simulink model "MotorXploer"  (R2024b)
settings: Solver=FixedStepAuto  StartTime=0.0  StopTime=inf  FixedStep=0.001  RelTol=1e-3
undefined symbols (not defined in the file): Blocking, LF, Non
libraries: hdlsllib x5, amg_usbconverter_n_connect_lib x3
settings Model: Creator=beamk  LastModifiedBy=pongn

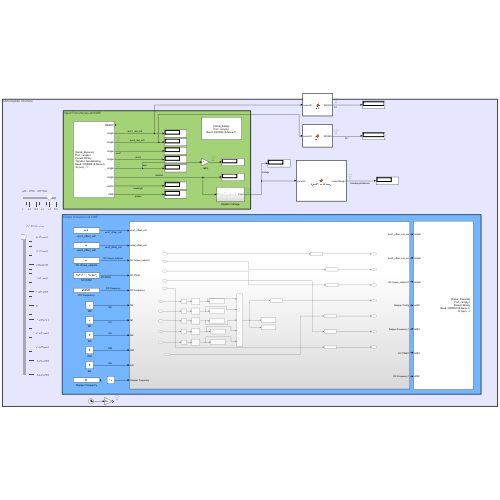
[thumbnail: Simulink's stored preview of the top-level diagram]
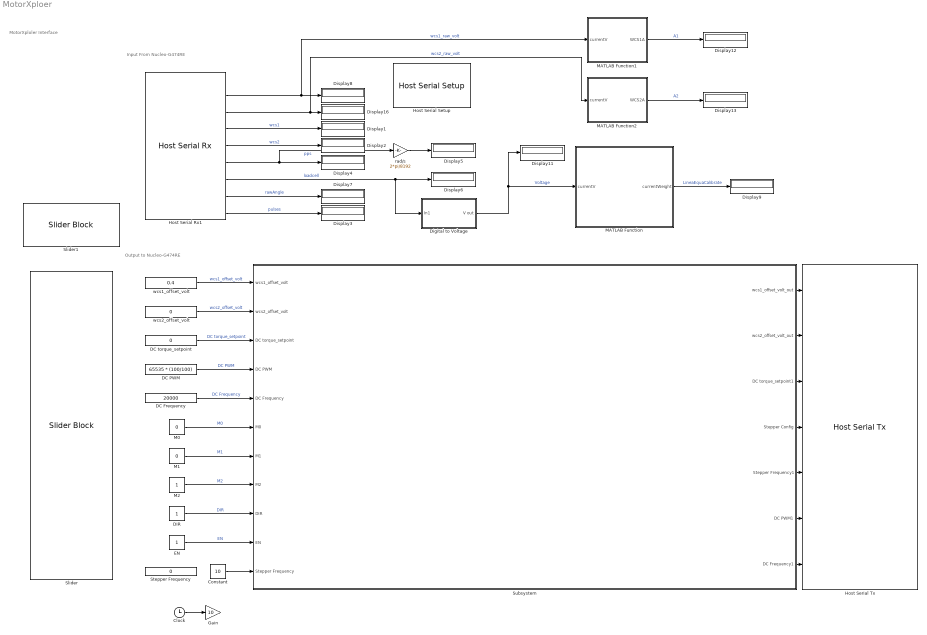
== system MotorXploer ==
  note: Output to Nucleo-G474RE
  note: Input From Nucleo-G474RE
  note: MotorXploler Interface
  Clock : Clock
  Constant : Constant  Value=10
  DC Frequency : Constant  Value=20000
  DC PWM : Constant  Value=65535 * (100/100)
  DC torque_setpoint : Constant  Value=0
  DIR : Constant  OutDataTypeStr=uint8
  Digital to Voltage : Subsystem
  Display{1..9,11..13,16} (13 alike) : Display
  EN : Constant  OutDataTypeStr=uint8
  Gain : Gain  Gain=10
  Host Serial Rx1 : amg_usbconverter_n_connect_lib/Host Serial Rx  conf=rx  port=<auto>  baudrate=2000000  databits=8  parity=None  stopbit=1  flowcontrol=None  transfer=Non-Blocking  timeout=5  packetmode=Binary  enableinitialvalues=off  initialvalues=[]  binheader='45'  binterminator='A'  porttype_double=0  porttype_single=6  porttype_int8=0  porttype_uint8=0  porttype_int16=0  porttype_uint16=1  porttype_int32=1  porttype_uint32=0  asciiformat='%f,%f,%d,%d'  rx_asciiterminator="LF (0x0A - \"\\n\")"  tx_asciiterminator="CRLF (0x0D 0x0A - \"\\r\\n\")"  sampletime=-1  enablecustomportlabel=off  cinputportlabel=0  coutputportlabel=A  portpinstr=0  blockid=HostSerialRx1  inputporttype=[]  inputportwidth=[]  inputportlabel={}  outputporttype=[3 1 1 1 1 1 1 5 6]  outputportwidth=[1 1 1 1 1 1 1 1 1]  outputportlabel={'READY','single','single','single','single','single','single','uint16','int32'}  compat=0  optionstring=[]  autoport='<empty>'
  Host Serial Setup : amg_usbconverter_n_connect_lib/Host Serial Setup  conf=setup  port=<auto>  baudrate=2000000  databits=8  parity=None  stopbit=1  flowcontrol=None  transfer=Blocking  timeout=2  packetmode=Binary  initialvalues=[]  binheader='7E 7E'  binterminator='03 03'  porttype_double=0  porttype_single=1  porttype_int8=0  porttype_uint8=0  porttype_int16=0  porttype_uint16=0  porttype_int32=0  porttype_uint32=2  asciiformat='%d %u %x'  rx_asciiterminator="CRLF (0x0D 0x0A - \"\\r\\n\")"  tx_asciiterminator="CRLF (0x0D 0x0A - \"\\r\\n\")"  sampletime=-1  enablecustomportlabel=off  cinputportlabel=0  coutputportlabel=A  portpinstr=0  blockid=HostSerialSetup  inputporttype=[]  inputportwidth=[]  inputportlabel={}  outputporttype=[]  outputportwidth=[]  outputportlabel={}  compat=0  optionstring=[]  autoport='<empty>'
  Host Serial Tx : amg_usbconverter_n_connect_lib/Host Serial Tx  conf=tx  port=<auto>  baudrate=2000000  databits=8  parity=None  stopbit=1  flowcontrol=None  transfer=Blocking  timeout=2  packetmode=Binary  initialvalues=[]  binheader='45'  binterminator='A'  porttype_double=0  porttype_single=3  porttype_int8=0  porttype_uint8=1  porttype_int16=0  porttype_uint16=0  porttype_int32=3  porttype_uint32=0  asciiformat='%d,%f'  rx_asciiterminator="CRLF (0x0D 0x0A - \"\\r\\n\")"  tx_asciiterminator="CRLF (0x0D 0x0A - \"\\r\\n\")"  sampletime=-1  enablecustomportlabel=off  cinputportlabel=0  coutputportlabel=A  portpinstr=0  blockid=HostSerialTx  inputporttype=[1 1 1 3 6 6 6]  inputportwidth=[1 1 1 1 1 1 1]  inputportlabel={'single','single','single','uint8','int32','int32','int32'}  outputporttype=[]  outputportwidth=[]  outputportlabel={}  compat=0  optionstring=[]  autoport='<empty>'
      settings: SourceProductName=aMG USB Converter N
  M0 : Constant  Value=0  OutDataTypeStr=uint8
  M1 : Constant  Value=0  OutDataTypeStr=uint8
  M2 : Constant  OutDataTypeStr=uint8
  MATLAB Function : MATLAB Function  TreatAsAtomicUnit=on
  MATLAB Function1 : MATLAB Function  TreatAsAtomicUnit=on
  MATLAB Function2 : MATLAB Function  TreatAsAtomicUnit=on
  Slider : SliderBlock  ScaleMin=-65535  ScaleMax=65535
  Slider1 : SliderBlock  ScaleMax=0.5
  Stepper Frequency : Constant  Value=0
  Subsystem : Subsystem
  rad/s : Gain  Gain=2*pi/8192
  wcs1_offset_volt : Constant  Value=0.4  OutDataTypeStr=single
  wcs2_offset_volt : Constant  Value=0  OutDataTypeStr=single
  wires:
  Host Serial Rx1/2 -> MATLAB Function1/1(currentV), Display8/1  "wcs1_raw_volt"
  Host Serial Rx1/3 -> MATLAB Function2/1(currentV), Display16/1  "wcs2_raw_volt"
  Host Serial Rx1/7 -> Digital to Voltage/1(In1), Display6/1  "loadcell"
  Host Serial Rx1/5 -> Display2/1  "wcs2"
  Host Serial Rx1/8 -> Display7/1  "rawAngle"
  rad/s/1 -> Display5/1
  Host Serial Rx1/6 -> Display4/1, rad/s/1  "pps"
  Host Serial Rx1/9 -> Display3/1  "pulses"
  wcs1_offset_volt/1 -> Subsystem/1(wcs1_offset_volt)  "wcs1_offset_volt"
  wcs2_offset_volt/1 -> Subsystem/2(wcs2_offset_volt)  "wcs2_offset_volt"
  DC torque_setpoint/1 -> Subsystem/3(DC torque_setpoint)  "DC torque_setpoint"
  DC Frequency/1 -> Subsystem/5(DC Frequency)  "DC Frequency"
  M0/1 -> Subsystem/6(M0)  "M0"
  M1/1 -> Subsystem/7(M1)  "M1"
  M2/1 -> Subsystem/8(M2)  "M2"
  DIR/1 -> Subsystem/9(DIR)  "DIR"
  EN/1 -> Subsystem/10(EN)  "EN"
  Subsystem/1(wcs1_offset_volt_out) -> Host Serial Tx/1
  Subsystem/2(wcs2_offset_volt_out) -> Host Serial Tx/2
  Subsystem/3(DC torque_setpoint1) -> Host Serial Tx/3
  Subsystem/4(Stepper Config) -> Host Serial Tx/4
  Subsystem/5(Stepper Frequency1) -> Host Serial Tx/5
  Subsystem/6(DC PWM1) -> Host Serial Tx/6
  Subsystem/7(DC Frequency1) -> Host Serial Tx/7
  Clock/1 -> Gain/1
  MATLAB Function/1(currentWeight) -> Display9/1  "LineaEquaCalibrate"
  Digital to Voltage/1(V out) -> Display11/1, MATLAB Function/1(currentV)  "Voltage"
  Host Serial Rx1/4 -> Display1/1  "wcs1"
  MATLAB Function1/1(WCS1A) -> Display12/1  "A1"
  MATLAB Function2/1(WCS2A) -> Display13/1  "A2"
  DC PWM/1 -> Subsystem/4(DC PWM)  "DC PWM"
  Constant/1 -> Subsystem/11(Stepper Frequency)

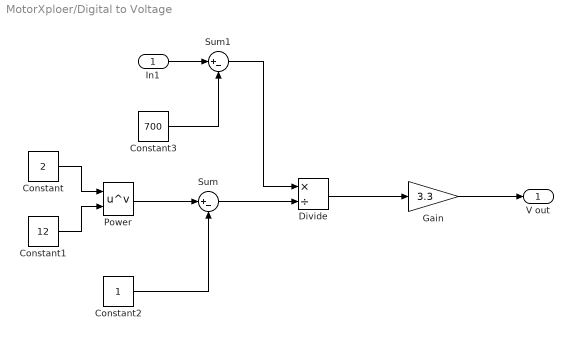
== system MotorXploer/Digital to Voltage ==
  In1 : Inport
  Constant : Constant  Value=2
  Constant1 : Constant  Value=12
  Constant2 : Constant
  Constant3 : Constant  Value=700
  Divide : Product  Inputs=*/
  Gain : Gain  Gain=3.3
  Power : Math  Operator=pow
  Sum : Sum  Inputs=|+-
  Sum1 : Sum  Inputs=|+-
  V out : Outport
  wires:
  Constant/1 -> Power/1
  Constant2/1 -> Sum/2
  Sum/1 -> Divide/2
  Power/1 -> Sum/1
  Divide/1 -> Gain/1
  Constant1/1 -> Power/2
  Gain/1 -> V out/1
  In1/1 -> Sum1/1
  Sum1/1 -> Divide/1
  Constant3/1 -> Sum1/2

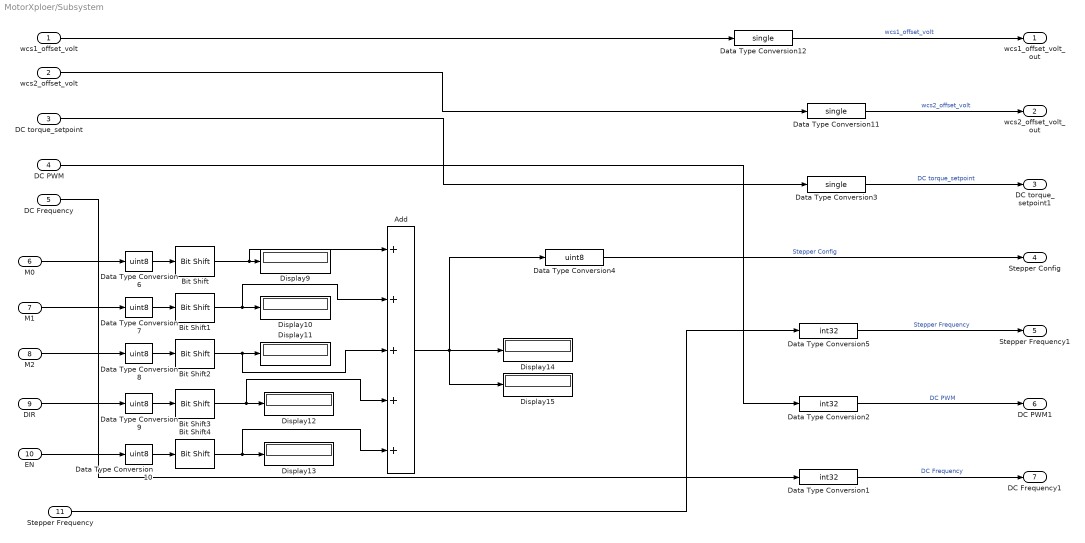
== system MotorXploer/Subsystem ==
  wcs1_offset_volt : Inport
  wcs2_offset_volt : Inport  Port=2
  DC torque_setpoint : Inport  Port=3
  DC PWM : Inport  Port=4
  DC Frequency : Inport  Port=5
  M0 : Inport  Port=6
  M1 : Inport  Port=7
  M2 : Inport  Port=8
  DIR : Inport  Port=9
  EN : Inport  Port=10
  Stepper Frequency : Inport  Port=11
  Add : Sum  Inputs=+++++
  Bit Shift : hdlsllib/Logic and Bit Operations/Bit Shift  mode=Shift Left Logical  N=4
  Bit Shift1 : hdlsllib/Logic and Bit Operations/Bit Shift  mode=Shift Left Logical  N=3
  Bit Shift2 : hdlsllib/Logic and Bit Operations/Bit Shift  mode=Shift Left Logical  N=2
  Bit Shift3 : hdlsllib/Logic and Bit Operations/Bit Shift  mode=Shift Left Logical  N=1
  Bit Shift4 : hdlsllib/Logic and Bit Operations/Bit Shift  mode=Shift Left Logical  N=0
  Data Type Conversion1 : DataTypeConversion  OutDataTypeStr=int32  SaturateOnIntegerOverflow=off  RndMeth=Floor
  Data Type Conversion{4,6..10} (6 alike) : DataTypeConversion  OutDataTypeStr=uint8  SaturateOnIntegerOverflow=off  RndMeth=Floor
  Data Type Conversion11 : DataTypeConversion  OutDataTypeStr=single  SaturateOnIntegerOverflow=off  RndMeth=Floor
  Data Type Conversion12 : DataTypeConversion  OutDataTypeStr=single  SaturateOnIntegerOverflow=off  RndMeth=Floor
  Data Type Conversion2 : DataTypeConversion  OutDataTypeStr=int32  SaturateOnIntegerOverflow=off  RndMeth=Floor
  Data Type Conversion3 : DataTypeConversion  OutDataTypeStr=single  SaturateOnIntegerOverflow=off  RndMeth=Floor
  Data Type Conversion5 : DataTypeConversion  OutDataTypeStr=int32  SaturateOnIntegerOverflow=off  RndMeth=Floor
  Display{9..15} (7 alike) : Display
      Display10 settings: Format=binary (Stored Integer)
      Display11 settings: Format=binary (Stored Integer)
      Display12 settings: Format=binary (Stored Integer)
      Display13 settings: Format=binary (Stored Integer)
      Display14 settings: Format=binary (Stored Integer)
      Display9 settings: Format=binary (Stored Integer)
  wcs1_offset_volt_out : Outport
  wcs2_offset_volt_out : Outport  Port=2
  DC torque_setpoint1 : Outport  Port=3
  Stepper Config : Outport  Port=4
  Stepper Frequency1 : Outport  Port=5
  DC PWM1 : Outport  Port=6
  DC Frequency1 : Outport  Port=7
  wires:
  Bit Shift/1 -> Display9/1, Add/1
  Data Type Conversion8/1 -> Bit Shift2/1
  EN/1 -> Data Type Conversion10/1
  Data Type Conversion6/1 -> Bit Shift/1
  DC torque_setpoint/1 -> Data Type Conversion3/1
  Data Type Conversion2/1 -> DC PWM1/1  "DC PWM"
  Data Type Conversion7/1 -> Bit Shift1/1
  Data Type Conversion10/1 -> Bit Shift4/1
  DC PWM/1 -> Data Type Conversion2/1
  Bit Shift3/1 -> Display12/1, Add/4
  Data Type Conversion12/1 -> wcs1_offset_volt_out/1  "wcs1_offset_volt"
  Add/1 -> Display15/1, Display14/1, Data Type Conversion4/1
  Bit Shift2/1 -> Display11/1, Add/3
  Stepper Frequency/1 -> Data Type Conversion5/1
  M1/1 -> Data Type Conversion7/1
  Bit Shift1/1 -> Display10/1, Add/2
  Bit Shift4/1 -> Display13/1, Add/5
  M0/1 -> Data Type Conversion6/1
  Data Type Conversion9/1 -> Bit Shift3/1
  Data Type Conversion11/1 -> wcs2_offset_volt_out/1  "wcs2_offset_volt"
  M2/1 -> Data Type Conversion8/1
  wcs1_offset_volt/1 -> Data Type Conversion12/1
  DC Frequency/1 -> Data Type Conversion1/1
  wcs2_offset_volt/1 -> Data Type Conversion11/1
  Data Type Conversion1/1 -> DC Frequency1/1  "DC Frequency"
  DIR/1 -> Data Type Conversion9/1
  Data Type Conversion4/1 -> Stepper Config/1  "Stepper Config"
  Data Type Conversion3/1 -> DC torque_setpoint1/1  "DC torque_setpoint"
  Data Type Conversion5/1 -> Stepper Frequency1/1  "Stepper Frequency"

== matlab function MotorXploer/MATLAB Function1 ==
  data: currentV input; WCS1A output
function WCS1A  = A1(currentV)
    WCS1A = (currentV * 30.5439545905890) - 64.2882337517370;
    end

== matlab function MotorXploer/MATLAB Function ==
  data: currentV input; currentWeight output
function currentWeight  = signalConditioning(currentV)
    currentWeight = (currentV * 2000) + 763;
    end

== matlab function MotorXploer/MATLAB Function2 ==
  data: currentV input; WCS2A output
function WCS2A  = A2(currentV)
    WCS2A = (currentV * 30.8323372813213) - 63.9102738237531;
    end
